simulink model "mandelbrot_fpga"  (R2019b)
settings: Solver=FixedStepDiscrete  StartTime=0.0  StopTime=33.5e-3  FixedStep=0.5*Ts  RelTol=1e-3  EnableMultiTasking=on
values from neighbouring files (symbols this model uses):
  BUTTON_CLOCK_DIV = 65536    [setup.m]
  BUTTON_DEBOUNCE = round(0.01/(Ts*BUTTON_CLOCK_DIV))    [setup.m]
  BUTTON_POLLING = round(0.01/(Ts*BUTTON_CLOCK_DIV))    [setup.m]
  LUT_BLUE = uint8(palette(:,3))    [generate_palette.m]
  LUT_GREEN = uint8(palette(:,2))    [generate_palette.m]
  LUT_RED = uint8(palette(:,1))    [generate_palette.m]
  MAX_ITERATIONS = 128    [setup.m]
  PIPELINE_SIZE = 64    [setup.m]
  PIXEL_TIME = 1    [config_screen_720p.m]    (also in config_screen_dummy.m)
  SEQUENTIAL_STEPS = 2    [setup.m]
  TRASLATION_FACTOR = 0.1    [setup.m]
  Ts = 1.35E-8    (= 1.35e-08)    [setup.m]
  VGA_HORIZONTAL_BACK_PORCH = 220    [config_screen_720p.m]    (also in config_screen_dummy.m = 1)
  VGA_HORIZONTAL_FRONT_PORCH = 110    [config_screen_720p.m]    (also in config_screen_dummy.m = 1)
  VGA_HORIZONTAL_RESOLUTION = 1280    [config_screen_720p.m]    (also in config_screen_dummy.m = 300)
  VGA_HORIZONTAL_SYNC = 40    [config_screen_720p.m]    (also in config_screen_dummy.m = 1)
  VGA_VERTICAL_BACK_PORCH = 20    [config_screen_720p.m]    (also in config_screen_dummy.m = 1)
  VGA_VERTICAL_FRONT_PORCH = 5    [config_screen_720p.m]    (also in config_screen_dummy.m = 1)
  VGA_VERTICAL_RESOLUTION = 720    [config_screen_720p.m]    (also in config_screen_dummy.m = 300)
  VGA_VERTICAL_SYNC = 5    [config_screen_720p.m]    (also in config_screen_dummy.m = 1)
  ZOOM_FACTOR = 0.98    [setup.m]
libraries: mandelbrot_library x13, hdlsllib x11, simulink x6, visionsinks x1
settings Model: OrderedModelArguments=off  Creator=sasselll  LastModifiedBy=lucas
settings SolverCC: ZeroCrossControl=DisableAll  PositivePriorityOrder=on  MinimalZcImpactIntegration=on
settings DataIOCC: SaveOutput=off  SignalLogging=off  DSMLogging=off
settings OptimizationCC: BlockReduction=off  ConditionallyExecuteInputs=off  DefaultParameterBehavior=Inlined  EnhancedBackFolding=on  PassReuseOutputArgsAs=Individual arguments  MaxStackSize=64  OptimizeBlockOrder=speed  DifferentSizesBufferReuse=on  UseRowMajorAlgorithm=on  OptimizationCustomize=off  EfficientTunableParamExpr=on
settings DebuggingCC: ReadBeforeWriteMsg=DisableAll  WriteAfterWriteMsg=DisableAll  WriteAfterReadMsg=DisableAll  AlgebraicLoopMsg=error  MultiTaskDSMMsg=none  ParameterTunabilityLossMsg=error
settings HardwareCC: ProdBitPerPointer=32  ProdBitPerSizeT=32  ProdBitPerPtrDiffT=32  ProdLargestAtomicFloat=None  ProdIntDivRoundTo=Undefined  ProdEndianess=Unspecified  ProdWordSize=32  ProdHWDeviceType=ASIC/FPGA->ASIC/FPGA  TargetBitPerPointer=64  TargetBitPerSizeT=64  TargetBitPerPtrDiffT=64  TargetLongLongMode=on  TargetIntDivRoundTo=Zero  TargetEndianess=LittleEndian  TargetWordSize=64  TargetHWDeviceType=Custom Processor->MATLAB Host Computer  ProdEqTarget=off  HardwareBoardFeatureSet=SoCBlockset
settings ModelReferenceCC: UpdateModelReferenceTargets=IfOutOfDate
settings SFSimCC: SFSimEcho=off  MATLABDynamicMemAlloc=off  CustomCodeUndefinedFunction=UseInterfaceOnly
settings RTWCC: SystemTargetFile=ert.tlc  TemplateMakefile=ert_default_tmf  GenerateReport=on  IncludeHyperlinkInReport=on  LaunchReport=on  GenerateTraceInfo=on  GenerateTraceReport=on  GenerateTraceReportSl=on  GenerateTraceReportSf=on  GenerateTraceReportEml=on
settings CodeAppCC: ForceParamTrailComments=on  IgnoreCustomStorageClasses=off  OperatorAnnotations=on  SimulinkDataObjDesc=on  SFDataObjDesc=on  InsertBlockDesc=on
settings ERTTargetCC: InlinedParameterPlacement=NonHierarchical  ERTCustomFileTemplate=example_file_process.tlc

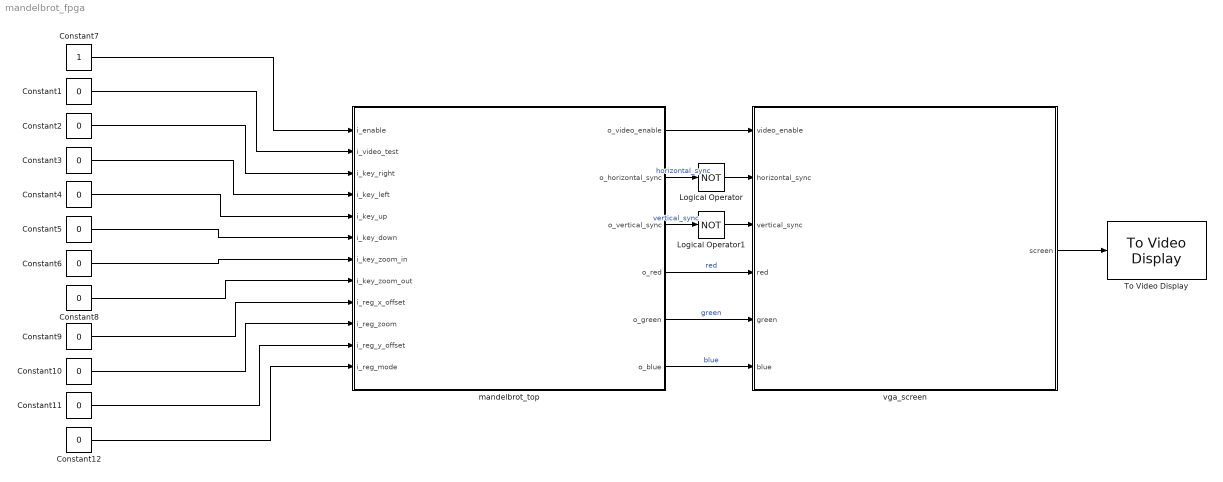
== system mandelbrot_fpga ==
  Constant{1..6,8..12} (11 alike) : Constant  Value=0  OutDataTypeStr=boolean  SampleTime=Ts
  Constant7 : Constant  OutDataTypeStr=boolean  SampleTime=Ts
  Logical Operator : Logic  Operator=NOT  IconShape=distinctive  AllPortsSameDT=off  OutDataTypeStr=boolean
  Logical Operator1 : Logic  Operator=NOT  IconShape=distinctive  AllPortsSameDT=off  OutDataTypeStr=boolean
  To Video Display : visionsinks/To Video Display  windowSizeMode=Normal  openAtMdlStart=on  fullScreen=off  videoWindowX=810  videoWindowY=390  saveWindowSize=off  videoWindowWidth=787  videoWindowHeight=554  inputColorFormat=RGB  inputType=Obsolete  imagePorts=One multidimensional signal  OutputDevice=On-screen video monitor  dataOrg=Column-major  isWindowOpen=off
      settings: SourceProductName=Computer Vision Toolbox
  mandelbrot_top : Subsystem
  vga_screen : Subsystem
  wires:
  Constant7/1 -> mandelbrot_top/1(i_enable)
  mandelbrot_top/4(o_red) -> vga_screen/4(red)  "red"
  mandelbrot_top/5(o_green) -> vga_screen/5(green)  "green"
  mandelbrot_top/6(o_blue) -> vga_screen/6(blue)  "blue"
  vga_screen/1(screen) -> To Video Display/1
  mandelbrot_top/1(o_video_enable) -> vga_screen/1("video_enable ")
  Constant1/1 -> mandelbrot_top/2(i_video_test)
  mandelbrot_top/2("o_horizontal_sync ") -> Logical Operator/1  "horizontal_sync"
  Logical Operator/1 -> vga_screen/2("horizontal_sync ")
  mandelbrot_top/3(o_vertical_sync) -> Logical Operator1/1  "vertical_sync"
  Logical Operator1/1 -> vga_screen/3("vertical_sync ")
  Constant2/1 -> mandelbrot_top/3(i_key_right)
  Constant3/1 -> mandelbrot_top/4(i_key_left)
  Constant4/1 -> mandelbrot_top/5(i_key_up)
  Constant5/1 -> mandelbrot_top/6(i_key_down)
  Constant6/1 -> mandelbrot_top/7(i_key_zoom_in)
  Constant8/1 -> mandelbrot_top/8(i_key_zoom_out)
  Constant9/1 -> mandelbrot_top/9(i_reg_x_offset)
  Constant10/1 -> mandelbrot_top/10(i_reg_zoom)
  Constant11/1 -> mandelbrot_top/11(i_reg_y_offset)
  Constant12/1 -> mandelbrot_top/12(i_reg_mode)

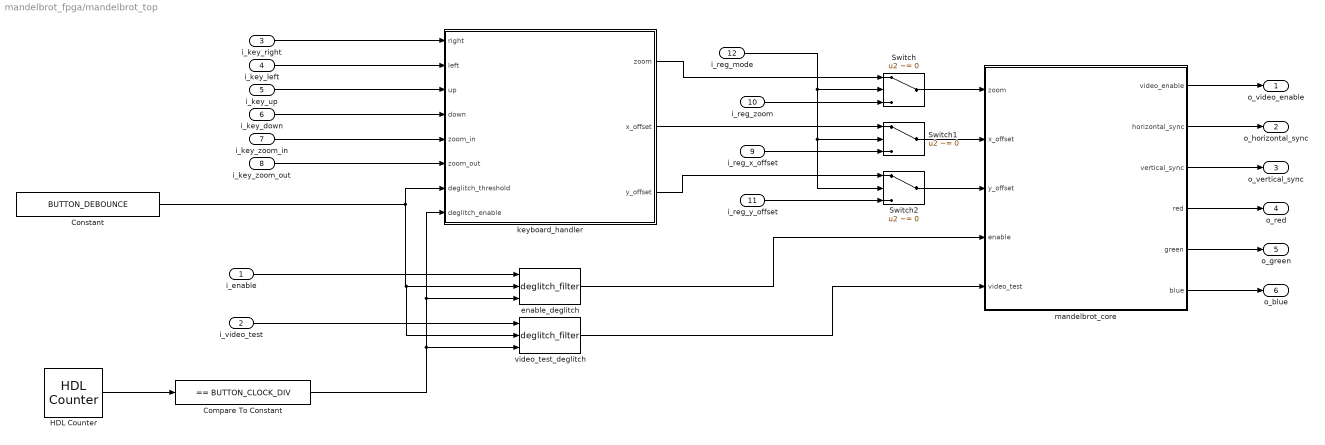
== system mandelbrot_fpga/mandelbrot_top ==
  i_enable : Inport
  i_video_test : Inport  Port=2
  i_key_right : Inport  Port=3
  i_key_left : Inport  Port=4
  i_key_up : Inport  Port=5
  i_key_down : Inport  Port=6
  i_key_zoom_in : Inport  Port=7
  i_key_zoom_out : Inport  Port=8
  i_reg_x_offset : Inport  Port=9
  i_reg_zoom : Inport  Port=10
  i_reg_y_offset : Inport  Port=11
  i_reg_mode : Inport  Port=12
  Compare To Constant : simulink/Logic and Bit Operations/Compare To Constant  relop===  const=BUTTON_CLOCK_DIV  OutDataTypeStr=boolean
  Constant : Constant  Value=BUTTON_DEBOUNCE  OutDataTypeStr=uint8  SampleTime=-1
  HDL Counter : hdlsllib/Sources/HDL Counter  CountType=Count limited  CountInit=0  CountStep=1  CountMax=BUTTON_CLOCK_DIV  CountFromType=Initial value  CountFrom=0  CountResetPort=off  CountLoadPort=off  CountEnbPort=off  CountDirPort=off  CountDataType=Unsigned  CountWordLen=17  CountFracLen=0  CountSampTime=Ts
      settings: SourceProductName=Simulink
  Switch : Switch  Criteria=u2 ~= 0
  Switch1 : Switch  Criteria=u2 ~= 0
  Switch2 : Switch  Criteria=u2 ~= 0
  enable_deglitch : mandelbrot_library/deglitch_filter  SystemSampleTime=-1  Latency=0  AutoFrameSizeCalculation=off
  "keyboard_handler " : Subsystem
  mandelbrot_core : Subsystem
  video_test_deglitch : mandelbrot_library/deglitch_filter  SystemSampleTime=-1  Latency=0  AutoFrameSizeCalculation=off
  o_video_enable : Outport  VectorParamsAs1DForOutWhenUnconnected=off
  "o_horizontal_sync " : Outport  Port=2  VectorParamsAs1DForOutWhenUnconnected=off
  o_vertical_sync : Outport  Port=3  VectorParamsAs1DForOutWhenUnconnected=off
  o_red : Outport  Port=4  VectorParamsAs1DForOutWhenUnconnected=off
  o_green : Outport  Port=5  VectorParamsAs1DForOutWhenUnconnected=off
  o_blue : Outport  Port=6  VectorParamsAs1DForOutWhenUnconnected=off
  wires:
  mandelbrot_core/3(vertical_sync) -> o_vertical_sync/1
  mandelbrot_core/4(red) -> o_red/1
  mandelbrot_core/2(horizontal_sync) -> "o_horizontal_sync "/1
  mandelbrot_core/6(blue) -> o_blue/1
  mandelbrot_core/5(green) -> o_green/1
  i_enable/1 -> enable_deglitch/1
  enable_deglitch/1 -> mandelbrot_core/4(enable)
  mandelbrot_core/1(video_enable) -> o_video_enable/1
  video_test_deglitch/1 -> mandelbrot_core/5(video_test)
  i_video_test/1 -> video_test_deglitch/1
  i_key_right/1 -> "keyboard_handler "/1(right)
  i_key_left/1 -> "keyboard_handler "/2(left)
  i_key_up/1 -> "keyboard_handler "/3(up)
  i_key_down/1 -> "keyboard_handler "/4(down)
  i_key_zoom_in/1 -> "keyboard_handler "/5(zoom_in)
  i_key_zoom_out/1 -> "keyboard_handler "/6(zoom_out)
  Constant/1 -> video_test_deglitch/2, enable_deglitch/2, "keyboard_handler "/7("deglitch_threshold ")
  HDL Counter/1 -> Compare To Constant/1
  Compare To Constant/1 -> video_test_deglitch/3, enable_deglitch/3, "keyboard_handler "/8(deglitch_enable)
  "keyboard_handler "/1(zoom) -> Switch/1
  Switch/1 -> mandelbrot_core/1(zoom)
  Switch1/1 -> mandelbrot_core/2("x_offset ")
  "keyboard_handler "/2(x_offset) -> Switch1/1
  Switch2/1 -> mandelbrot_core/3("y_offset ")
  "keyboard_handler "/3(y_offset) -> Switch2/1
  i_reg_y_offset/1 -> Switch2/3
  i_reg_x_offset/1 -> Switch1/3
  i_reg_zoom/1 -> Switch/3
  i_reg_mode/1 -> Switch2/2, Switch1/2, Switch/2

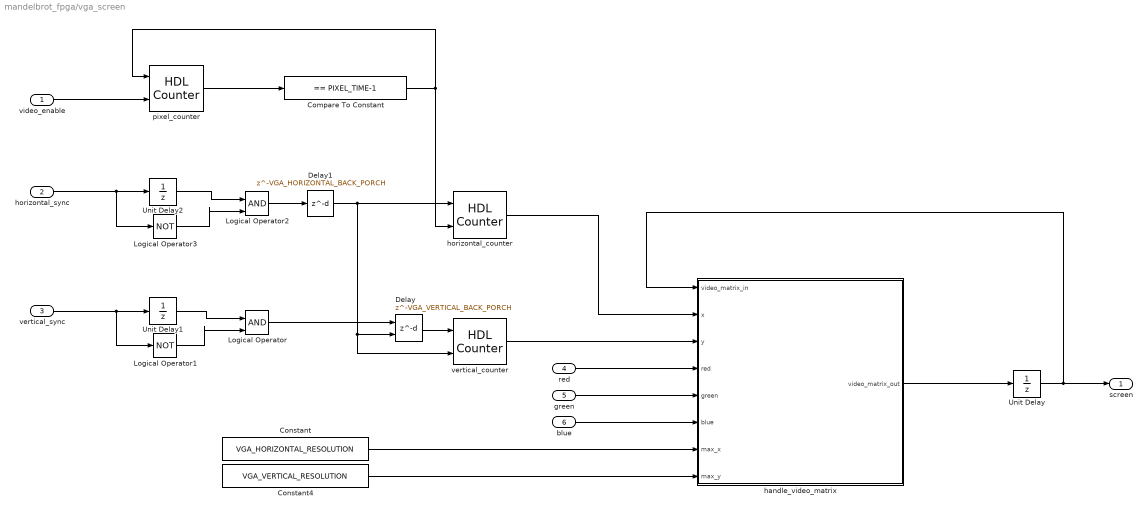
== system mandelbrot_fpga/vga_screen ==
  "video_enable " : Inport
  "horizontal_sync " : Inport  Port=2
  "vertical_sync " : Inport  Port=3
  red : Inport  Port=4
  green : Inport  Port=5
  blue : Inport  Port=6
  Compare To Constant : simulink/Logic and Bit Operations/Compare To Constant  relop===  const=PIXEL_TIME-1  OutDataTypeStr=boolean
  Constant : Constant  Value=VGA_HORIZONTAL_RESOLUTION  SampleTime=-1
  Constant4 : Constant  Value=VGA_VERTICAL_RESOLUTION  SampleTime=-1
  Delay : Delay  DelayLength=VGA_VERTICAL_BACK_PORCH  InitialCondition=0  ShowEnablePort=on
      settings: InputPortMap=u0,e6
  Delay1 : Delay  DelayLength=VGA_HORIZONTAL_BACK_PORCH  InitialCondition=0
  Logical Operator : Logic  IconShape=distinctive  AllPortsSameDT=off  OutDataTypeStr=boolean
  Logical Operator1 : Logic  Operator=NOT  IconShape=distinctive  AllPortsSameDT=off  OutDataTypeStr=boolean
  Logical Operator2 : Logic  IconShape=distinctive  AllPortsSameDT=off  OutDataTypeStr=boolean
  Logical Operator3 : Logic  Operator=NOT  IconShape=distinctive  AllPortsSameDT=off  OutDataTypeStr=boolean
  Unit Delay : UnitDelay  SampleTime=-1  HasFrameUpgradeWarning=on
  Unit Delay1 : UnitDelay  SampleTime=-1  HasFrameUpgradeWarning=on
  Unit Delay2 : UnitDelay  SampleTime=-1  HasFrameUpgradeWarning=on
  handle_video_matrix : MATLAB Function  TreatAsAtomicUnit=on
  horizontal_counter : hdlsllib/Sources/HDL Counter  CountType=Free running  CountInit=1  CountStep=1  CountMax=25  CountFromType=Initial value  CountFrom=1  CountResetPort=on  CountLoadPort=off  CountEnbPort=on  CountDirPort=off  CountDataType=Unsigned  CountWordLen=16  CountFracLen=0  CountSampTime=1
      settings: SourceProductName=Simulink
  "pixel_counter " : hdlsllib/Sources/HDL Counter  CountType=Free running  CountInit=0  CountStep=1  CountMax=PIXEL_TIME  CountFromType=Initial value  CountFrom=0  CountResetPort=on  CountLoadPort=off  CountEnbPort=on  CountDirPort=off  CountDataType=Unsigned  CountWordLen=8  CountFracLen=0  CountSampTime=Ts
      settings: SourceProductName=Simulink
  vertical_counter : hdlsllib/Sources/HDL Counter  CountType=Free running  CountInit=1  CountStep=1  CountMax=25  CountFromType=Initial value  CountFrom=1  CountResetPort=on  CountLoadPort=off  CountEnbPort=on  CountDirPort=off  CountDataType=Unsigned  CountWordLen=16  CountFracLen=0  CountSampTime=1
      settings: SourceProductName=Simulink
  screen : Outport  PortDimensions=[VGA_VERTICAL_RESOLUTION VGA_HORIZONTAL_RESOLUTION 3]  VectorParamsAs1DForOutWhenUnconnected=off
  wires:
  "pixel_counter "/1 -> Compare To Constant/1
  "horizontal_sync "/1 -> Logical Operator3/1, Unit Delay2/1
  Compare To Constant/1 -> "pixel_counter "/1, horizontal_counter/2
  Unit Delay/1 -> screen/1, handle_video_matrix/1(video_matrix_in)
  red/1 -> handle_video_matrix/4(red)
  green/1 -> handle_video_matrix/5(green)
  vertical_counter/1 -> handle_video_matrix/3(y)
  handle_video_matrix/1(video_matrix_out) -> Unit Delay/1
  "vertical_sync "/1 -> Logical Operator1/1, Unit Delay1/1
  blue/1 -> handle_video_matrix/6(blue)
  horizontal_counter/1 -> handle_video_matrix/2(x)
  Constant/1 -> handle_video_matrix/7(max_x)
  Constant4/1 -> handle_video_matrix/8(max_y)
  Unit Delay2/1 -> Logical Operator2/1
  Logical Operator3/1 -> Logical Operator2/2
  Logical Operator1/1 -> Logical Operator/2
  Unit Delay1/1 -> Logical Operator/1
  Logical Operator/1 -> Delay/1
  Delay/1 -> vertical_counter/1
  Logical Operator2/1 -> Delay1/1
  Delay1/1 -> horizontal_counter/1, Delay/2, vertical_counter/2
  "video_enable "/1 -> "pixel_counter "/2

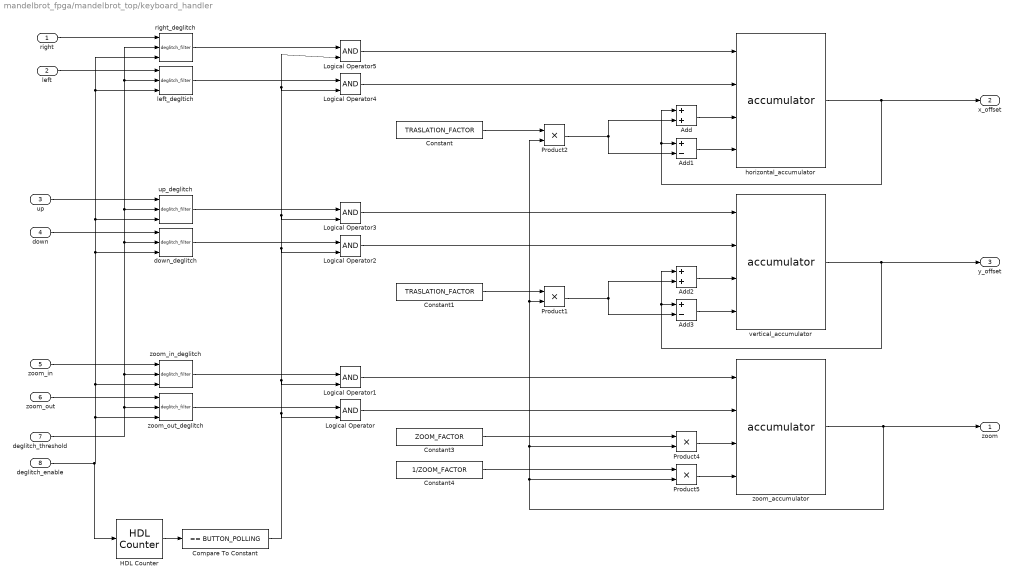
== system mandelbrot_fpga/mandelbrot_top/keyboard_handler  ==
  right : Inport
  left : Inport  Port=2
  up : Inport  Port=3
  down : Inport  Port=4
  zoom_in : Inport  Port=5
  zoom_out : Inport  Port=6
  "deglitch_threshold " : Inport  Port=7
  deglitch_enable : Inport  Port=8
  Add : Sum
  Add1 : Sum  Inputs=+-
  Add2 : Sum
  Add3 : Sum  Inputs=+-  OutDataTypeStr=Inherit: Same as first input
  Compare To Constant : simulink/Logic and Bit Operations/Compare To Constant  relop===  const=BUTTON_POLLING  OutDataTypeStr=boolean
  Constant : Constant  Value=TRASLATION_FACTOR  OutDataTypeStr=Inherit: Inherit via back propagation  SampleTime=-1
  Constant1 : Constant  Value=TRASLATION_FACTOR  OutDataTypeStr=Z_BUS_TYPE  SampleTime=-1
  Constant3 : Constant  Value=ZOOM_FACTOR  OutDataTypeStr=Z_BUS_TYPE  SampleTime=-1
  Constant4 : Constant  Value=1/ZOOM_FACTOR  OutDataTypeStr=Z_BUS_TYPE  SampleTime=-1
  HDL Counter : hdlsllib/Sources/HDL Counter  CountType=Count limited  CountInit=0  CountStep=1  CountMax=BUTTON_POLLING  CountFromType=Initial value  CountFrom=0  CountResetPort=off  CountLoadPort=off  CountEnbPort=on  CountDirPort=off  CountDataType=Unsigned  CountWordLen=8  CountFracLen=0  CountSampTime=1
      settings: SourceProductName=Simulink
  Logical Operator{,1..5} (6 alike) : Logic  IconShape=distinctive  AllPortsSameDT=off  OutDataTypeStr=boolean
  Product{1..2,4..5} (4 alike) : Product  OutDataTypeStr=Inherit: Same as first input
  "down_deglitch " : mandelbrot_library/deglitch_filter  SystemSampleTime=-1  Latency=0  AutoFrameSizeCalculation=off
  horizontal_accumulator : mandelbrot_library/accumulator  SystemSampleTime=-1  Latency=0  AutoFrameSizeCalculation=off
  left_degltich : mandelbrot_library/deglitch_filter  SystemSampleTime=-1  Latency=0  AutoFrameSizeCalculation=off
  right_deglitch : mandelbrot_library/deglitch_filter  SystemSampleTime=-1  Latency=0  AutoFrameSizeCalculation=off
  up_deglitch : mandelbrot_library/deglitch_filter  SystemSampleTime=-1  Latency=0  AutoFrameSizeCalculation=off
  vertical_accumulator : mandelbrot_library/accumulator  SystemSampleTime=-1  Latency=0  AutoFrameSizeCalculation=off
  zoom_accumulator : mandelbrot_library/accumulator  SystemSampleTime=-1  Latency=0  AutoFrameSizeCalculation=off
      link override Unit Delay Enabled Synchronous: InitialCondition=1
  zoom_in_deglitch : mandelbrot_library/deglitch_filter  SystemSampleTime=-1  Latency=0  AutoFrameSizeCalculation=off
  zoom_out_deglitch : mandelbrot_library/deglitch_filter  SystemSampleTime=-1  Latency=0  AutoFrameSizeCalculation=off
  zoom : Outport  OutDataTypeStr=Z_BUS_TYPE
  x_offset : Outport  Port=2  OutDataTypeStr=Z_BUS_TYPE
  y_offset : Outport  Port=3  OutDataTypeStr=Z_BUS_TYPE
  wires:
  Add/1 -> horizontal_accumulator/3
  Add1/1 -> horizontal_accumulator/4
  Add2/1 -> vertical_accumulator/3
  Logical Operator/1 -> zoom_accumulator/2
  Logical Operator1/1 -> zoom_accumulator/1
  Logical Operator3/1 -> vertical_accumulator/1
  Logical Operator2/1 -> vertical_accumulator/2
  Logical Operator5/1 -> horizontal_accumulator/1
  Logical Operator4/1 -> horizontal_accumulator/2
  zoom_in_deglitch/1 -> Logical Operator1/1
  zoom_out_deglitch/1 -> Logical Operator/1
  zoom_in/1 -> zoom_in_deglitch/1
  zoom_out/1 -> zoom_out_deglitch/1
  up_deglitch/1 -> Logical Operator3/1
  "down_deglitch "/1 -> Logical Operator2/1
  up/1 -> up_deglitch/1
  down/1 -> "down_deglitch "/1
  right/1 -> right_deglitch/1
  left/1 -> left_degltich/1
  left_degltich/1 -> Logical Operator4/1
  right_deglitch/1 -> Logical Operator5/1
  "deglitch_threshold "/1 -> "down_deglitch "/2, right_deglitch/2, left_degltich/2, up_deglitch/2, zoom_in_deglitch/2, zoom_out_deglitch/2
  HDL Counter/1 -> Compare To Constant/1
  Compare To Constant/1 -> Logical Operator4/2, Logical Operator5/2, Logical Operator3/2, Logical Operator2/2, Logical Operator1/2, Logical Operator/2
  Product5/1 -> zoom_accumulator/4
  Product4/1 -> zoom_accumulator/3
  Constant3/1 -> Product4/1
  Constant4/1 -> Product5/1
  deglitch_enable/1 -> HDL Counter/1, zoom_out_deglitch/3, up_deglitch/3, right_deglitch/3, left_degltich/3, "down_deglitch "/3, zoom_in_deglitch/3
  horizontal_accumulator/1 -> x_offset/1, Add1/1, Add/1
  vertical_accumulator/1 -> y_offset/1, Add3/1, Add2/1
  zoom_accumulator/1 -> zoom/1, Product5/2, Product4/2, Product2/2, Product1/2
  Add3/1 -> vertical_accumulator/4
  Product1/1 -> Add3/2, Add2/2
  Constant1/1 -> Product1/1
  Product2/1 -> Add/2, Add1/2
  Constant/1 -> Product2/1

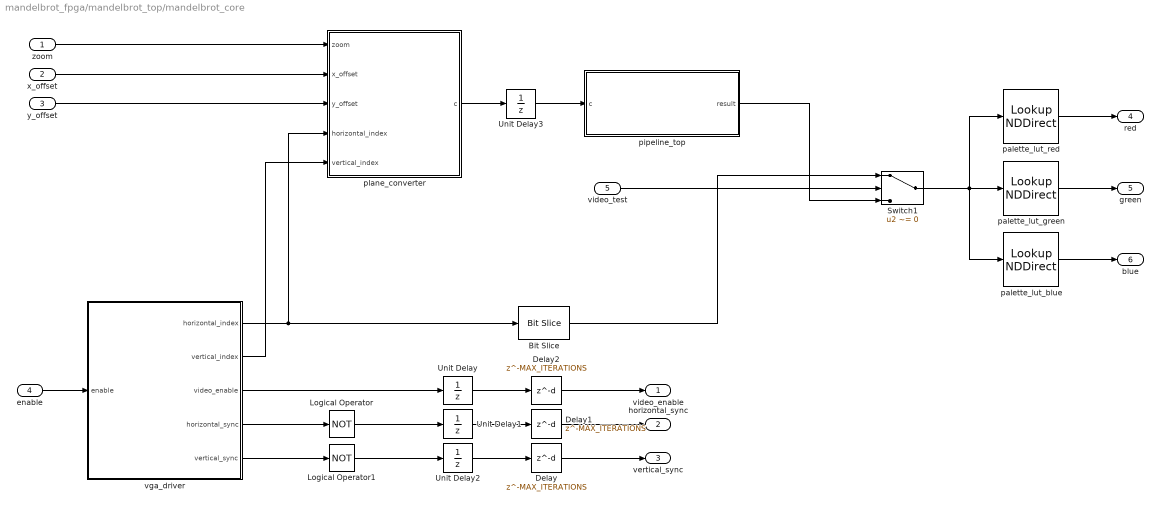
== system mandelbrot_fpga/mandelbrot_top/mandelbrot_core ==
  zoom : Inport
  "x_offset " : Inport  Port=2
  "y_offset " : Inport  Port=3
  enable : Inport  Port=4
  video_test : Inport  Port=5
  Bit Slice : hdlsllib/Logic and Bit Operations/Bit Slice  lidx=6  ridx=0
      settings: SourceProductName=Simulink  SourceProductBaseCode=SL
  Delay : Delay  DelayLength=MAX_ITERATIONS
  Delay1 : Delay  DelayLength=MAX_ITERATIONS
  Delay2 : Delay  DelayLength=MAX_ITERATIONS
  Logical Operator : Logic  Operator=NOT  IconShape=distinctive  AllPortsSameDT=off  OutDataTypeStr=boolean
  Logical Operator1 : Logic  Operator=NOT  IconShape=distinctive  AllPortsSameDT=off  OutDataTypeStr=boolean
  Switch1 : Switch  Criteria=u2 ~= 0
  Unit Delay{,1..3} (4 alike) : UnitDelay  SampleTime=-1  HasFrameUpgradeWarning=on
  "palette_lut_blue " : LookupNDDirect  NumberOfTableDimensions=1  Table=LUT_BLUE  DiagnosticForOutOfRangeInput=Error
  "palette_lut_green " : LookupNDDirect  NumberOfTableDimensions=1  Table=LUT_GREEN  DiagnosticForOutOfRangeInput=Error
  "palette_lut_red " : LookupNDDirect  NumberOfTableDimensions=1  Table=LUT_RED  DiagnosticForOutOfRangeInput=Error
  pipeline_top : Subsystem
  "plane_converter " : Subsystem
  vga_driver : Subsystem
  video_enable : Outport  VectorParamsAs1DForOutWhenUnconnected=off
  horizontal_sync : Outport  Port=2  VectorParamsAs1DForOutWhenUnconnected=off
  vertical_sync : Outport  Port=3  VectorParamsAs1DForOutWhenUnconnected=off
  red : Outport  Port=4  VectorParamsAs1DForOutWhenUnconnected=off
  green : Outport  Port=5  VectorParamsAs1DForOutWhenUnconnected=off
  blue : Outport  Port=6  VectorParamsAs1DForOutWhenUnconnected=off
  wires:
  vga_driver/1(horizontal_index) -> Bit Slice/1, "plane_converter "/4("horizontal_index ")
  "x_offset "/1 -> "plane_converter "/2("x_offset ")
  "y_offset "/1 -> "plane_converter "/3("y_offset ")
  enable/1 -> vga_driver/1("enable ")
  vga_driver/2(vertical_index) -> "plane_converter "/5("vertical_index ")
  zoom/1 -> "plane_converter "/1(zoom)
  "palette_lut_red "/1 -> red/1
  "palette_lut_green "/1 -> green/1
  "palette_lut_blue "/1 -> blue/1
  vga_driver/4(horizontal_sync) -> Logical Operator/1
  vga_driver/5("vertical_sync ") -> Logical Operator1/1
  Switch1/1 -> "palette_lut_blue "/1, "palette_lut_red "/1, "palette_lut_green "/1
  video_test/1 -> Switch1/2
  "plane_converter "/1(c) -> Unit Delay3/1
  pipeline_top/1(result) -> Switch1/3
  Bit Slice/1 -> Switch1/1
  Logical Operator1/1 -> Unit Delay2/1
  Delay/1 -> vertical_sync/1
  Logical Operator/1 -> Unit Delay1/1
  Delay1/1 -> horizontal_sync/1
  vga_driver/3("video_enable ") -> Unit Delay/1
  Delay2/1 -> video_enable/1
  Unit Delay/1 -> Delay2/1
  Unit Delay1/1 -> Delay1/1
  Unit Delay2/1 -> Delay/1
  Unit Delay3/1 -> pipeline_top/1(c)

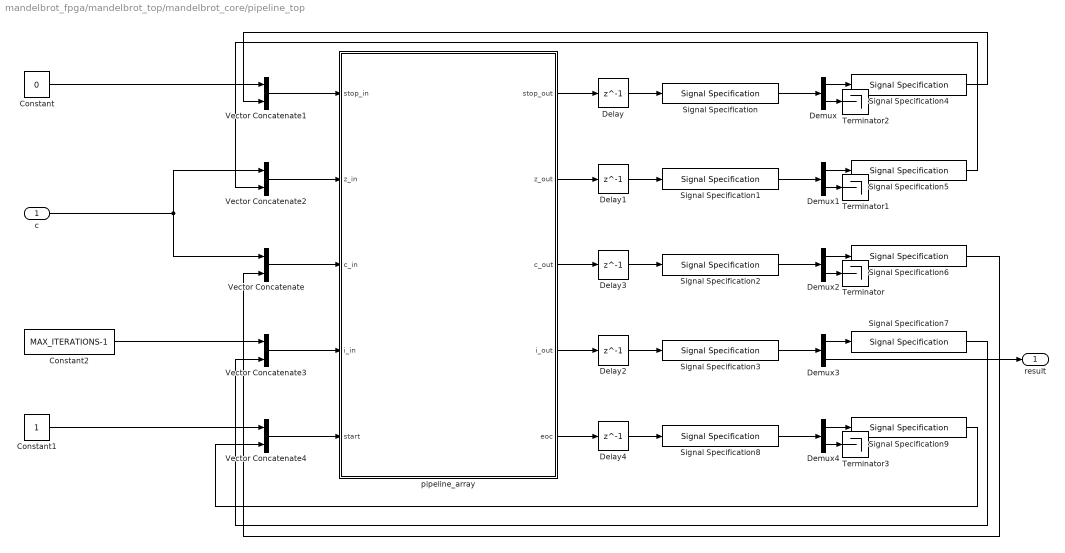
== system mandelbrot_fpga/mandelbrot_top/mandelbrot_core/pipeline_top ==
  c : Inport
  Constant : Constant  Value=0  OutDataTypeStr=boolean  SampleTime=-1
  Constant1 : Constant  OutDataTypeStr=boolean  SampleTime=-1
  Constant2 : Constant  Value=MAX_ITERATIONS-1  OutDataTypeStr=fixdt(0,7)  SampleTime=-1
  Delay{,1..4} (5 alike) : Delay  DelayLength=1  InitialCondition=0  SampleTime=Ts
  Demux{,1..4} (5 alike) : Demux  Outputs=2
  Signal Specification{,1..3,8} (5 alike) : SignalSpecification  Dimensions=PIPELINE_SIZE
  Signal Specification{4..7,9} (5 alike) : SignalSpecification  Dimensions=PIPELINE_SIZE-1
  Terminator{,1..3} (4 alike) : Terminator
  Vector Concatenate{,1..4} (5 alike) : Concatenate
  pipeline_array : Subsystem
  result : Outport  VectorParamsAs1DForOutWhenUnconnected=off
  wires:
  pipeline_array/4(i_out) -> Delay2/1
  pipeline_array/2(z_out) -> Delay1/1
  pipeline_array/1(stop_out) -> Delay/1
  pipeline_array/3(c_out) -> Delay3/1
  Vector Concatenate/1 -> pipeline_array/3(c_in)
  Delay/1 -> Signal Specification/1
  Delay1/1 -> Signal Specification1/1
  Delay3/1 -> Signal Specification2/1
  Delay2/1 -> Signal Specification3/1
  Signal Specification/1 -> Demux/1
  Demux/1 -> Signal Specification4/1
  Signal Specification1/1 -> Demux1/1
  Demux1/1 -> Signal Specification5/1
  Signal Specification3/1 -> Demux3/1
  Demux3/1 -> Signal Specification7/1
  Signal Specification2/1 -> Demux2/1
  Demux2/1 -> Signal Specification6/1
  Vector Concatenate1/1 -> pipeline_array/1(stop_in)
  Vector Concatenate2/1 -> pipeline_array/2(z_in)
  Constant/1 -> Vector Concatenate1/1
  Signal Specification4/1 -> Vector Concatenate1/2
  Signal Specification5/1 -> Vector Concatenate2/2
  Signal Specification6/1 -> Vector Concatenate/2
  Signal Specification7/1 -> Vector Concatenate3/2
  Vector Concatenate3/1 -> pipeline_array/4(i_in)
  Constant2/1 -> Vector Concatenate3/1
  Demux2/2 -> Terminator/1
  Demux3/2 -> result/1
  Demux/2 -> Terminator2/1
  Demux1/2 -> Terminator1/1
  c/1 -> Vector Concatenate/1, Vector Concatenate2/1
  Constant1/1 -> Vector Concatenate4/1
  Signal Specification9/1 -> Vector Concatenate4/2
  Vector Concatenate4/1 -> pipeline_array/5(start)
  Signal Specification8/1 -> Demux4/1
  Demux4/2 -> Terminator3/1
  Demux4/1 -> Signal Specification9/1
  Delay4/1 -> Signal Specification8/1
  pipeline_array/5(eoc) -> Delay4/1

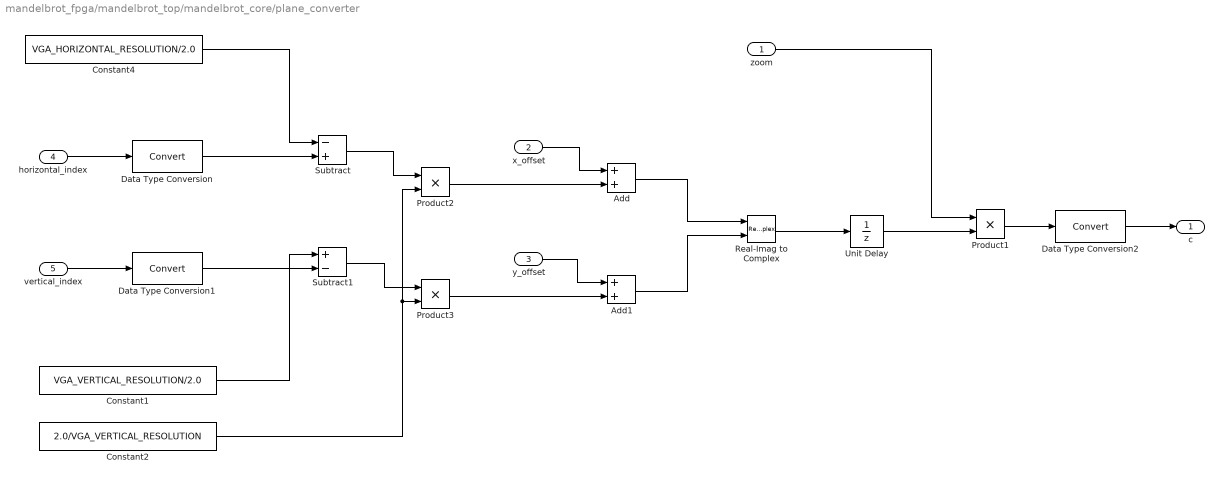
== system mandelbrot_fpga/mandelbrot_top/mandelbrot_core/plane_converter  ==
  zoom : Inport
  "x_offset " : Inport  Port=2
  "y_offset " : Inport  Port=3
  "horizontal_index " : Inport  Port=4
  "vertical_index " : Inport  Port=5
  Add : Sum
  Add1 : Sum
  Constant1 : Constant  Value=VGA_VERTICAL_RESOLUTION/2.0  OutDataTypeStr=fixdt(1,12,0)  SampleTime=-1
  Constant2 : Constant  Value=2.0/VGA_VERTICAL_RESOLUTION  OutDataTypeStr=Z_BUS_TYPE  SampleTime=-1
  Constant4 : Constant  Value=VGA_HORIZONTAL_RESOLUTION/2.0  OutDataTypeStr=fixdt(1,12,0)  SampleTime=-1
  Data Type Conversion : DataTypeConversion
  Data Type Conversion1 : DataTypeConversion
  Data Type Conversion2 : DataTypeConversion
  Product1 : Product
  Product2 : Product
  Product3 : Product
  Real-Imag to Complex : RealImagToComplex
  Subtract : Sum  Inputs=-+
  Subtract1 : Sum  Inputs=+-
  Unit Delay : UnitDelay  SampleTime=-1  HasFrameUpgradeWarning=on
  c : Outport  OutDataTypeStr=Z_BUS_TYPE  VectorParamsAs1DForOutWhenUnconnected=off
  wires:
  Subtract1/1 -> Product3/1
  Add/1 -> Real-Imag to Complex/1
  "y_offset "/1 -> Add1/1
  Add1/1 -> Real-Imag to Complex/2
  Constant4/1 -> Subtract/1
  "x_offset "/1 -> Add/1
  "horizontal_index "/1 -> Data Type Conversion/1
  Data Type Conversion/1 -> Subtract/2
  "vertical_index "/1 -> Data Type Conversion1/1
  Data Type Conversion1/1 -> Subtract1/2
  Subtract/1 -> Product2/1
  zoom/1 -> Product1/1
  Constant1/1 -> Subtract1/1
  Constant2/1 -> Product3/2, Product2/2
  Product2/1 -> Add/2
  Product3/1 -> Add1/2
  Data Type Conversion2/1 -> c/1
  Product1/1 -> Data Type Conversion2/1
  Real-Imag to Complex/1 -> Unit Delay/1
  Unit Delay/1 -> Product1/2

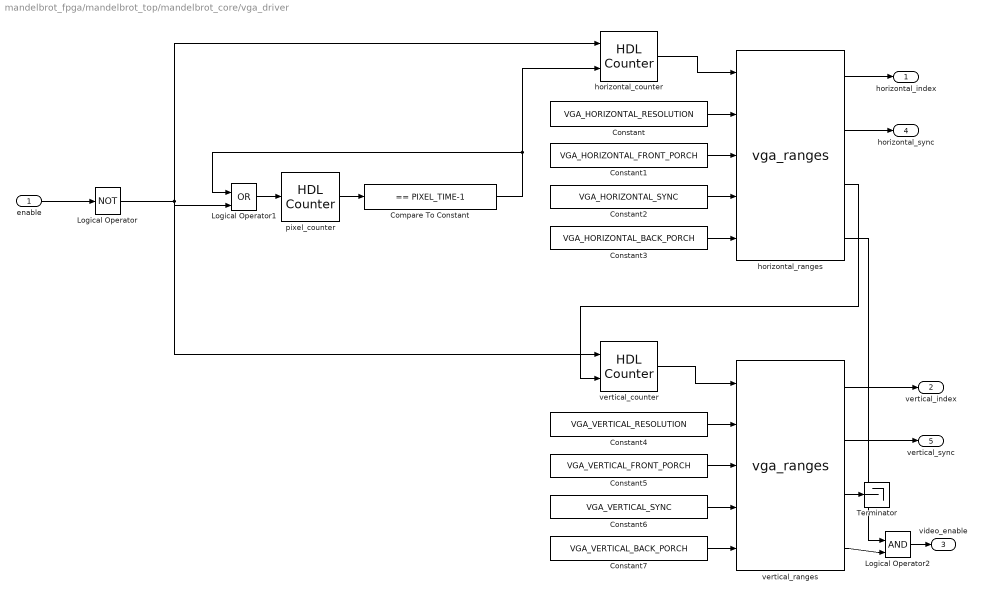
== system mandelbrot_fpga/mandelbrot_top/mandelbrot_core/vga_driver ==
  "enable " : Inport
  Compare To Constant : simulink/Logic and Bit Operations/Compare To Constant  relop===  const=PIXEL_TIME-1  OutDataTypeStr=boolean
  Constant : Constant  Value=VGA_HORIZONTAL_RESOLUTION  OutDataTypeStr=uint16  SampleTime=-1
  Constant1 : Constant  Value=VGA_HORIZONTAL_FRONT_PORCH  OutDataTypeStr=uint16  SampleTime=-1
  Constant2 : Constant  Value=VGA_HORIZONTAL_SYNC  OutDataTypeStr=uint16  SampleTime=-1
  Constant3 : Constant  Value=VGA_HORIZONTAL_BACK_PORCH  OutDataTypeStr=uint16  SampleTime=-1
  Constant4 : Constant  Value=VGA_VERTICAL_RESOLUTION  OutDataTypeStr=uint16  SampleTime=-1
  Constant5 : Constant  Value=VGA_VERTICAL_FRONT_PORCH  OutDataTypeStr=uint16  SampleTime=-1
  Constant6 : Constant  Value=VGA_VERTICAL_SYNC  OutDataTypeStr=uint16  SampleTime=-1
  Constant7 : Constant  Value=VGA_VERTICAL_BACK_PORCH  OutDataTypeStr=uint16  SampleTime=-1
  Logical Operator : Logic  Operator=NOT  IconShape=distinctive  AllPortsSameDT=off  OutDataTypeStr=boolean
  Logical Operator1 : Logic  Operator=OR  IconShape=distinctive  AllPortsSameDT=off  OutDataTypeStr=boolean
  Logical Operator2 : Logic  IconShape=distinctive  AllPortsSameDT=off  OutDataTypeStr=boolean
  Terminator : Terminator
  horizontal_counter : hdlsllib/Sources/HDL Counter  CountType=Count limited  CountInit=0  CountStep=1  CountMax=VGA_HORIZONTAL_RESOLUTION+VGA_HORIZONTAL_FRONT_PORCH+VGA_HORIZONTAL_SYNC+VGA_HORIZONTAL_BACK_PORCH-1  CountFromType=Initial value  CountFrom=0  CountResetPort=on  CountLoadPort=off  CountEnbPort=on  CountDirPort=off  CountDataType=Unsigned  CountWordLen=16  CountFracLen=0  CountSampTime=1
      settings: SourceProductName=Simulink
  horizontal_ranges : mandelbrot_library/vga_ranges  SystemSampleTime=-1  Latency=0  AutoFrameSizeCalculation=off
  "pixel_counter " : hdlsllib/Sources/HDL Counter  CountType=Count limited  CountInit=0  CountStep=1  CountMax=PIXEL_TIME  CountFromType=Initial value  CountFrom=0  CountResetPort=on  CountLoadPort=off  CountEnbPort=off  CountDirPort=off  CountDataType=Unsigned  CountWordLen=8  CountFracLen=0  CountSampTime=Ts
      settings: SourceProductName=Simulink
  "vertical_counter " : hdlsllib/Sources/HDL Counter  CountType=Count limited  CountInit=0  CountStep=1  CountMax=VGA_VERTICAL_RESOLUTION+VGA_VERTICAL_FRONT_PORCH+VGA_VERTICAL_SYNC+VGA_VERTICAL_BACK_PORCH-1  CountFromType=Initial value  CountFrom=0  CountResetPort=on  CountLoadPort=off  CountEnbPort=on  CountDirPort=off  CountDataType=Unsigned  CountWordLen=16  CountFracLen=0  CountSampTime=1
      settings: SourceProductName=Simulink
  "vertical_ranges " : mandelbrot_library/vga_ranges  SystemSampleTime=-1  Latency=0  AutoFrameSizeCalculation=off
  horizontal_index : Outport  VectorParamsAs1DForOutWhenUnconnected=off
  vertical_index : Outport  Port=2  VectorParamsAs1DForOutWhenUnconnected=off
  "video_enable " : Outport  Port=3  OutDataTypeStr=boolean  VectorParamsAs1DForOutWhenUnconnected=off
  horizontal_sync : Outport  Port=4  OutDataTypeStr=boolean  VectorParamsAs1DForOutWhenUnconnected=off
  "vertical_sync " : Outport  Port=5  OutDataTypeStr=boolean  VectorParamsAs1DForOutWhenUnconnected=off
  wires:
  horizontal_counter/1 -> horizontal_ranges/1
  Constant/1 -> horizontal_ranges/2
  Constant1/1 -> horizontal_ranges/3
  Constant2/1 -> horizontal_ranges/4
  Constant3/1 -> horizontal_ranges/5
  horizontal_ranges/2 -> horizontal_sync/1
  Constant5/1 -> "vertical_ranges "/3
  "vertical_ranges "/1 -> vertical_index/1
  Constant4/1 -> "vertical_ranges "/2
  Constant6/1 -> "vertical_ranges "/4
  "vertical_counter "/1 -> "vertical_ranges "/1
  Constant7/1 -> "vertical_ranges "/5
  "vertical_ranges "/2 -> "vertical_sync "/1
  horizontal_ranges/3 -> "vertical_counter "/2
  "enable "/1 -> Logical Operator/1
  Logical Operator/1 -> Logical Operator1/2, horizontal_counter/1, "vertical_counter "/1
  "vertical_ranges "/3 -> Terminator/1
  "pixel_counter "/1 -> Compare To Constant/1
  Compare To Constant/1 -> horizontal_counter/2, Logical Operator1/1
  Logical Operator1/1 -> "pixel_counter "/1
  "vertical_ranges "/4 -> Logical Operator2/2
  horizontal_ranges/4 -> Logical Operator2/1
  Logical Operator2/1 -> "video_enable "/1
  horizontal_ranges/1 -> horizontal_index/1

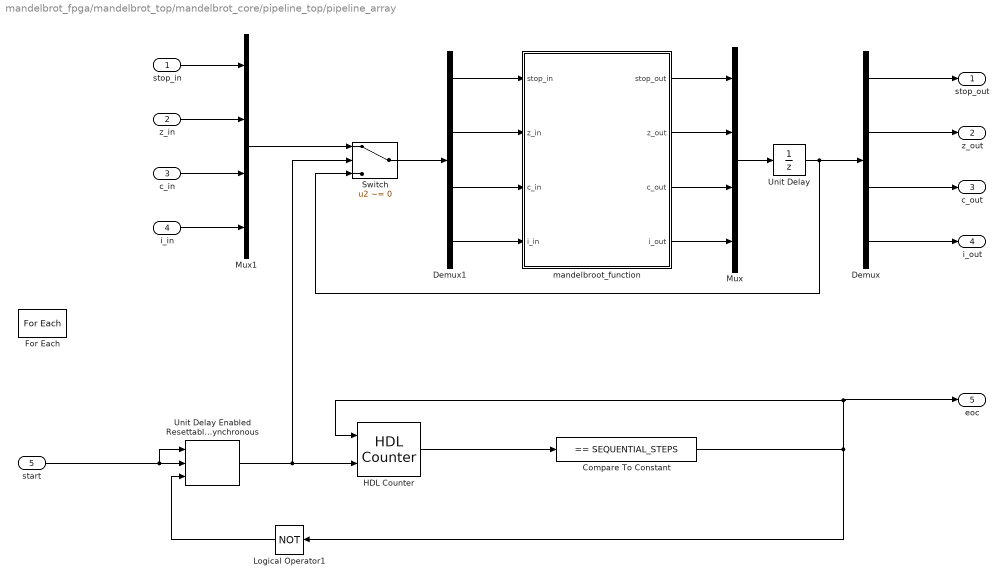
== system mandelbrot_fpga/mandelbrot_top/mandelbrot_core/pipeline_top/pipeline_array ==
  stop_in : Inport  Partition=on  PartitionDimension=1  PartitionWidth=1  PartitionOffset=0
  z_in : Inport  Port=2  Partition=on  PartitionDimension=1  PartitionWidth=1  PartitionOffset=0
  c_in : Inport  Port=3  Partition=on  PartitionDimension=1  PartitionWidth=1  PartitionOffset=0
  i_in : Inport  Port=4  Partition=on  PartitionDimension=1  PartitionWidth=1  PartitionOffset=0
  start : Inport  Port=5  Partition=on  PartitionDimension=1  PartitionWidth=1  PartitionOffset=0
  Compare To Constant : simulink/Logic and Bit Operations/Compare To Constant  relop===  const=SEQUENTIAL_STEPS  OutDataTypeStr=boolean
  Demux : Demux
  Demux1 : Demux
  For Each : ForEach  DisableCoverage=on
  HDL Counter : hdlsllib/Sources/HDL Counter  CountType=Count limited  CountInit=0  CountStep=1  CountMax=SEQUENTIAL_STEPS  CountFromType=Initial value  CountFrom=0  CountResetPort=on  CountLoadPort=off  CountEnbPort=on  CountDirPort=off  CountDataType=Unsigned  CountWordLen=2  CountFracLen=0  CountSampTime=1
      settings: SourceProductName=Simulink
  Logical Operator1 : Logic  Operator=NOT  IconShape=distinctive  AllPortsSameDT=off  OutDataTypeStr=boolean
  Mux : Mux
  Mux1 : Mux
  Switch : Switch  Criteria=u2 ~= 0
  Unit Delay : UnitDelay  SampleTime=-1  HasFrameUpgradeWarning=on
  Unit Delay Enabled Resettable Synchronous : hdlsllib/Discrete/Unit Delay Enabled Resettable Synchronous  InitialCondition=0.0  SampleTime=-1
      settings: SourceProductName=Simulink  SourceProductBaseCode=SL
  mandelbroot_function : Subsystem
  stop_out : Outport  ConcatenationDimension=1  VectorParamsAs1DForOutWhenUnconnected=off
  z_out : Outport  Port=2  ConcatenationDimension=1  VectorParamsAs1DForOutWhenUnconnected=off
  c_out : Outport  Port=3  ConcatenationDimension=1  VectorParamsAs1DForOutWhenUnconnected=off
  i_out : Outport  Port=4  ConcatenationDimension=1  VectorParamsAs1DForOutWhenUnconnected=off
  eoc : Outport  Port=5  ConcatenationDimension=1  VectorParamsAs1DForOutWhenUnconnected=off
  wires:
  Demux/2 -> z_out/1
  Demux/1 -> stop_out/1
  start/1 -> Unit Delay Enabled Resettable Synchronous/1, Unit Delay Enabled Resettable Synchronous/2
  i_in/1 -> Mux1/4
  stop_in/1 -> Mux1/1
  c_in/1 -> Mux1/3
  Switch/1 -> Demux1/1
  Demux/4 -> i_out/1
  Demux1/2 -> mandelbroot_function/2(z_in)
  Demux1/1 -> mandelbroot_function/1(stop_in)
  Demux1/4 -> mandelbroot_function/4(i_in)
  mandelbroot_function/1(stop_out) -> Mux/1
  Logical Operator1/1 -> Unit Delay Enabled Resettable Synchronous/3
  mandelbroot_function/3(c_out) -> Mux/3
  Demux1/3 -> mandelbroot_function/3(c_in)
  HDL Counter/1 -> Compare To Constant/1
  Unit Delay Enabled Resettable Synchronous/1 -> HDL Counter/2, Switch/2
  Mux1/1 -> Switch/1
  z_in/1 -> Mux1/2
  Compare To Constant/1 -> eoc/1, HDL Counter/1, Logical Operator1/1
  mandelbroot_function/4(i_out) -> Mux/4
  Demux/3 -> c_out/1
  Unit Delay/1 -> Switch/3, Demux/1
  Mux/1 -> Unit Delay/1
  mandelbroot_function/2(z_out) -> Mux/2

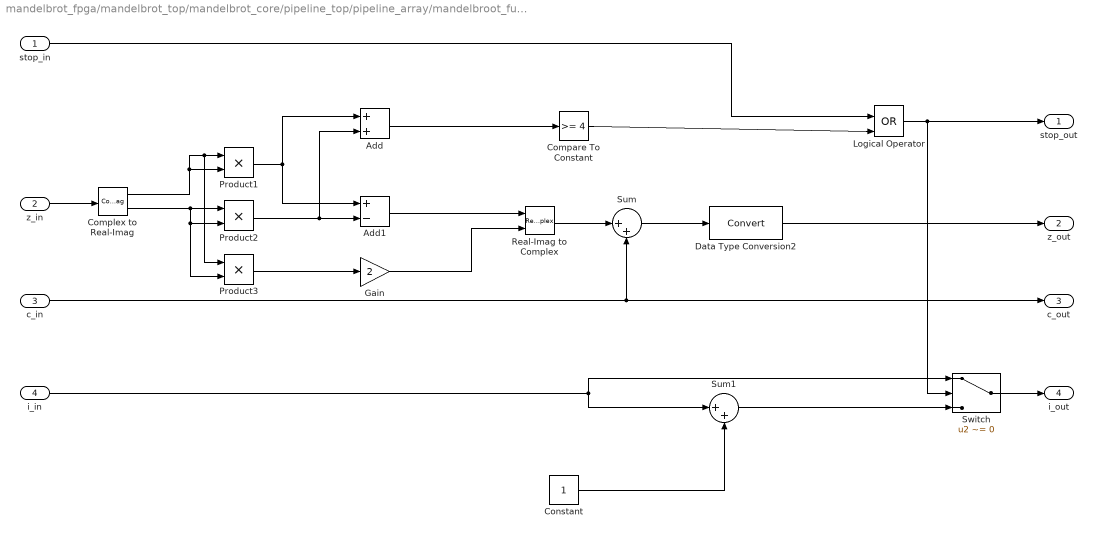
== system mandelbrot_fpga/mandelbrot_top/mandelbrot_core/pipeline_top/pipeline_array/mandelbroot_function ==
  stop_in : Inport
  z_in : Inport  Port=2
  c_in : Inport  Port=3
  i_in : Inport  Port=4
  Add : Sum
  Add1 : Sum  Inputs=+-  OutDataTypeStr=Inherit: Same as first input
  Compare To Constant : simulink/Logic and Bit Operations/Compare To Constant  relop=>=  const=4  OutDataTypeStr=boolean
  Complex to Real-Imag : ComplexToRealImag
  Constant : Constant  OutDataTypeStr=uint8  SampleTime=-1
  Data Type Conversion2 : DataTypeConversion
  Gain : Gain  Gain=2  OutDataTypeStr=Inherit: Same as input  ParamDataTypeStr=Inherit: Same as input
  Logical Operator : Logic  Operator=OR  IconShape=distinctive  AllPortsSameDT=off  OutDataTypeStr=boolean
  Product1 : Product
  Product2 : Product
  Product3 : Product
  Real-Imag to Complex : RealImagToComplex
  Sum : Sum  Inputs=|++  OutDataTypeStr=Inherit: Same as first input
  Sum1 : Sum  Inputs=|++
  Switch : Switch  Criteria=u2 ~= 0
  stop_out : Outport  VectorParamsAs1DForOutWhenUnconnected=off
  z_out : Outport  Port=2  VectorParamsAs1DForOutWhenUnconnected=off
  c_out : Outport  Port=3  VectorParamsAs1DForOutWhenUnconnected=off
  i_out : Outport  Port=4  VectorParamsAs1DForOutWhenUnconnected=off
  wires:
  Complex to Real-Imag/1 -> Product3/1, Product1/1, Product1/2
  Gain/1 -> Real-Imag to Complex/2
  Add1/1 -> Real-Imag to Complex/1
  Data Type Conversion2/1 -> z_out/1
  Complex to Real-Imag/2 -> Product3/2, Product2/2, Product2/1
  Product1/1 -> Add1/1, Add/1
  Product2/1 -> Add1/2, Add/2
  Logical Operator/1 -> stop_out/1, Switch/2
  Add/1 -> Compare To Constant/1
  i_in/1 -> Switch/1, Sum1/1
  Real-Imag to Complex/1 -> Sum/1
  c_in/1 -> c_out/1, Sum/2
  stop_in/1 -> Logical Operator/1
  z_in/1 -> Complex to Real-Imag/1
  Product3/1 -> Gain/1
  Constant/1 -> Sum1/2
  Sum/1 -> Data Type Conversion2/1
  Compare To Constant/1 -> Logical Operator/2
  Switch/1 -> i_out/1
  Sum1/1 -> Switch/3

== matlab function mandelbrot_fpga/vga_screen/handle_video_matrix ==
  data: video_matrix_in input; video_matrix_out output; x input; y input; red input; green input; blue input; max_x input; max_y input
function video_matrix_out = handle_video_matrix(video_matrix_in, x, y, red, green, blue, max_x, max_y)
%#codegen

temp = video_matrix_in;
if x <= max_x && y <= max_y 
    temp(y, x, :) = [double(red)/255.0 double(green)/255.0 double(blue)/255.0];
end
video_matrix_out = temp;
